simulink model "Syetem08"  (R2022b)
settings: Solver=ode45  StartTime=0.0  StopTime=Time  FixedStep=0.0001  RelTol=1e-6
values from neighbouring files (symbols this model uses):
  C1 = 2*M1*Wn1*zeta    [Syetem08_Parameters.m]
  C2 = 2*M2*Wn2*zeta    [Syetem08_Parameters.m]
  C3 = 2*M3*Wn3*zeta    [Syetem08_Parameters.m]
  dCD11 = 6.5*u    (= 6.5e-06)    [Syetem08_Parameters.m]
  dCD12 = 7.5*u    (= 7.5e-06)    [Syetem08_Parameters.m]
  dCD13 = 17*u    (= 1.7e-05)    [Syetem08_Parameters.m]
  dCD31 = dCD11    (= 6.5e-06)    [Syetem08_Parameters.m]
  dCD32 = dCD12    (= 7.5e-06)    [Syetem08_Parameters.m]
  dCD33 = dCD13    (= 1.7e-05)    [Syetem08_Parameters.m]
  epsilon = 8.854*u^2    (= 8.854e-12)    [Syetem08_Parameters.m]
  FAmp = -6*2*18*g    (= -2118.96)    [Syetem08_Parameters.m]
  g = 9.81    [Syetem08_Parameters.m]
  gCD1 = 5*u    (= 5e-06)    [Syetem08_Parameters.m]
  gCD3 = gCD1    (= 5e-06)    [Syetem08_Parameters.m]
  gppL1 = (14+.4)*u    (= 1.44e-05)    [Syetem08_Parameters.m]
  gppL12 = (20.5+.4+0.7+inaccuracy)*u    (= 2.21e-05)    [Syetem08_Parameters.m]
  gppL2 = (7+.4+inaccuracy)*u    (= 7.9e-06)    [Syetem08_Parameters.m]
  gppL3 = (7+.4-1.1+.1)*u    (= 6.4e-06)    [Syetem08_Parameters.m]
  gppL32 = (20.5+.4+0.7+inaccuracy)*u    (= 2.21e-05)    [Syetem08_Parameters.m]
  gppU1 = (7+.4-1.1+.2)*u    (= 6.5e-06)    [Syetem08_Parameters.m]
  gppU12 = (11.5+.4-0.7-inaccuracy)*u    (= 1.07e-05)    [Syetem08_Parameters.m]
  gppU2 = (7+.4-inaccuracy)*u    (= 6.9e-06)    [Syetem08_Parameters.m]
  gppU3 = (14+.4)*u    (= 1.44e-05)    [Syetem08_Parameters.m]
  gppU32 = (11.5+.4-0.7-inaccuracy)*u    (= 1.07e-05)    [Syetem08_Parameters.m]
  InputRatio = 0.814    [Syetem08_Parameters.m]
  K1 = 3*Kfactor*.9    (= 2.7)    [Syetem08_Parameters.m]
  K2 = 3*Kfactor*0.9    (= 2.7)    [Syetem08_Parameters.m]
  K3 = 3*Kfactor*.9    (= 2.7)    [Syetem08_Parameters.m]
  L1 = (215-.4)*u    (= 0.0002146)    [Syetem08_Parameters.m]
  L12 = (310-.4)*u    (= 0.0003096)    [Syetem08_Parameters.m]
  L2 = (215-.4)*u    (= 0.0002146)    [Syetem08_Parameters.m]
  L3 = (215-.4)*u    (= 0.0002146)    [Syetem08_Parameters.m]
  L32 = (310-.4)*u    (= 0.0003096)    [Syetem08_Parameters.m]
  M1 = rho*Depth*58910*u^2*Mfactor    (= 1.97654832e-07)    [Syetem08_Parameters.m]
  M2 = rho*Depth*75513.66*u^2*Mfactor    (= 2.53363432032e-07)    [Syetem08_Parameters.m]
  M3 = M1    (= 1.97654832e-07)    [Syetem08_Parameters.m]
  N1 = 8    [Syetem08_Parameters.m]
  N12 = 6    [Syetem08_Parameters.m]
  N2 = 2*5    (= 10)    [Syetem08_Parameters.m]
  N3 = N1    (= 8)    [Syetem08_Parameters.m]
  N32 = 6    [Syetem08_Parameters.m]
  NCD1 = 25    [Syetem08_Parameters.m]
  NCD3 = NCD1    (= 25)    [Syetem08_Parameters.m]
  S1 = [-inf 4.4]*u    [Syetem08_Parameters.m]
  S2 = [-(4.9+inaccuracy) (4.9-inaccuracy)]*u    [Syetem08_Parameters.m]
  S3 = [-3.7 inf]*u    [Syetem08_Parameters.m]
  t1 = 50*u    (= 5e-05)    [Syetem08_Parameters.m]
  t2 = t1    (= 5e-05)    [Syetem08_Parameters.m]
  t3 = t1    (= 5e-05)    [Syetem08_Parameters.m]
  Vcd1 = Vm1    (= 8.5)    [Syetem08_Parameters.m]
  Vm1 = 8.5    [Syetem08_Parameters.m]
  Vm2 = 27.5    [Syetem08_Parameters.m]
  Vm3 = 8.6    [Syetem08_Parameters.m]
  Vpp1 = Vm1    (= 8.5)    [Syetem08_Parameters.m]
  Vpp2 = 0    [Syetem08_Parameters.m]
  Vpp3 = Vm3    (= 8.6)    [Syetem08_Parameters.m]
  wCD1 = 3.5*u    (= 3.5e-06)    [Syetem08_Parameters.m]
  WCD1 = 427.5*u    (= 0.0004275)    [Syetem08_Parameters.m]
  wCD3 = wCD1    (= 3.5e-06)    [Syetem08_Parameters.m]
  WCD3 = WCD1    (= 0.0004275)    [Syetem08_Parameters.m]
undefined symbols (not defined in the file or in its folder): sigbuilder_block
settings Model: Creator=mokour  LastModifiedBy=Megdadi
settings DataIOCC: SaveFormat=StructureWithTime
settings OptimizationCC: LifeSpan=inf
settings DebuggingCC: UnconnectedInputMsg=warning  UnconnectedOutputMsg=warning  UnconnectedLineMsg=warning  SFExecutionAtInitializationDiag=none  SFMachineParentedDataDiag=warning  ArithmeticOperatorsInVariantConditions=warning
settings HardwareCC: ProdBitPerSizeT=32  ProdBitPerPtrDiffT=32  ProdWordSize=32  ProdHWDeviceType=Specified
settings ModelReferenceCC: EnableRefExpFcnMdlSchedulingChecks=on
settings SFSimCC: CustomCodeUndefinedFunction=UseInterfaceOnly
settings RTWCC: DLArmComputeVersion=19.05
settings CodeAppCC: StateflowObjectComments=on

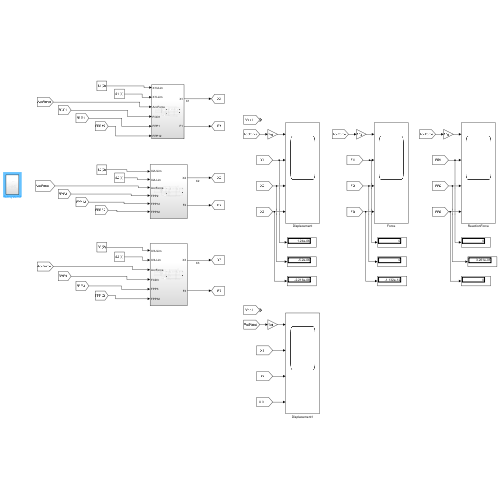
[thumbnail: Simulink's stored preview of the top-level diagram]
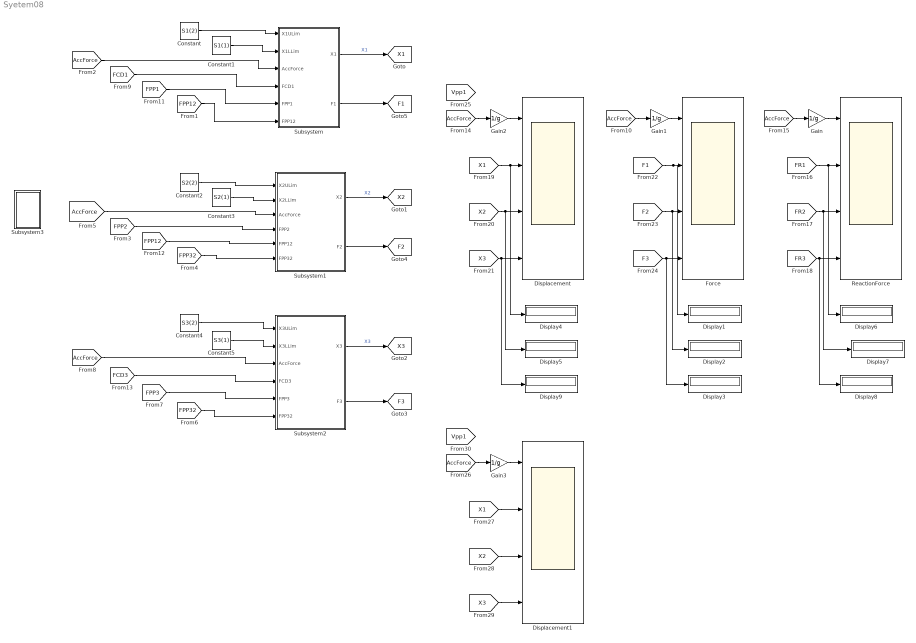
== system Syetem08 ==
  Constant : Constant  Value=S1(2)
  Constant1 : Constant  Value=S1(1)
  Constant2 : Constant  Value=S2(2)
  Constant3 : Constant  Value=S2(1)
  Constant4 : Constant  Value=S3(2)
  Constant5 : Constant  Value=S3(1)
  Displacement : Scope  NumInputPorts=4
  Displacement1 : Scope  NumInputPorts=4
  Display{1..9} (9 alike) : Display
  Force : Scope  NumInputPorts=4
  Gain{,1..3} (4 alike) : Gain  Gain=1/g
  ReactionForce : Scope  NumInputPorts=4
  Subsystem : Subsystem
  Subsystem1 : Subsystem
  Subsystem2 : Subsystem
  Subsystem3 : Subsystem
  tag scope: F1=global, F2=global, F3=global, X1=global, X2=global, X3=global
  wires:
  [FPP12] -> Subsystem/6(FPP12)
  [AccForce] -> Subsystem/3(AccForce)
  [FPP2] -> Subsystem1/4(FPP2)
  [FPP32] -> Subsystem1/6(FPP32)
  [AccForce] -> Subsystem1/3(AccForce)
  Subsystem1/1(X2) -> [X2]  "X2"
  Subsystem2/1(X3) -> [X3]  "X3"
  [FCD1] -> Subsystem/4(FCD1)
  [FPP1] -> Subsystem/5(FPP1)
  [FPP12] -> Subsystem1/5(FPP12)
  [FPP3] -> Subsystem2/5(FPP3)
  [FCD3] -> Subsystem2/4(FCD3)
  [AccForce] -> Subsystem2/3(AccForce)
  [FPP32] -> Subsystem2/6(FPP32)
  Subsystem2/2(F3) -> [F3]
  Subsystem/2(F1) -> [F1]
  Subsystem1/2(F2) -> [F2]
  Constant1/1 -> Subsystem/2(X1LLim)
  Constant/1 -> Subsystem/1(X1ULim)
  Constant3/1 -> Subsystem1/2(X2LLim)
  Constant2/1 -> Subsystem1/1(X2ULim)
  Constant4/1 -> Subsystem2/1(X3ULim)
  Constant5/1 -> Subsystem2/2(X3LLim)
  Gain/1 -> ReactionForce/1
  [FR1] -> ReactionForce/2, Display6/1
  [FR2] -> ReactionForce/3, Display7/1
  [FR3] -> ReactionForce/4, Display8/1
  Subsystem/1(X1) -> [X1]  "X1"
  [F3] -> Force/4, Display3/1
  [F2] -> Force/3, Display2/1
  [F1] -> Display1/1, Force/2
  [X1] -> Display4/1, Displacement/2
  [X2] -> Display5/1, Displacement/3
  [X3] -> Displacement/4, Display9/1
  [AccForce] -> Gain/1
  [AccForce] -> Gain1/1
  Gain1/1 -> Force/1
  [AccForce] -> Gain2/1
  Gain2/1 -> Displacement/1
  Gain3/1 -> Displacement1/1
  [AccForce] -> Gain3/1
  [X3] -> Displacement1/4
  [X2] -> Displacement1/3
  [X1] -> Displacement1/2

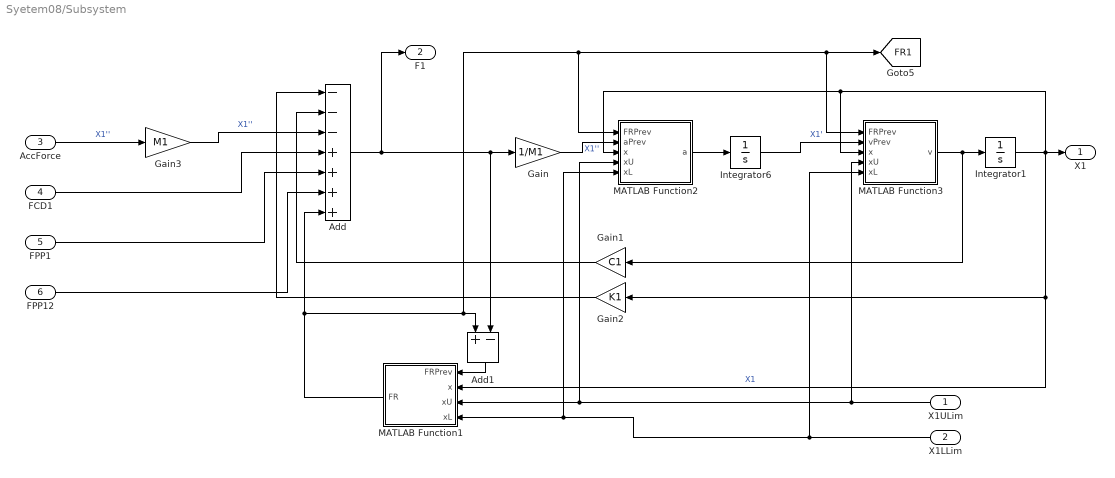
== system Syetem08/Subsystem ==
  X1ULim : Inport
  X1LLim : Inport  Port=2
  AccForce : Inport  Port=3
  FCD1 : Inport  Port=4
  FPP1 : Inport  Port=5
  FPP12 : Inport  Port=6
  Add : Sum  Inputs=---++++
  Add1 : Sum  Inputs=+-
  Gain : Gain  Gain=1/M1
  Gain1 : Gain  Gain=C1
  Gain2 : Gain  Gain=K1
  Gain3 : Gain  Gain=M1
  Integrator1 : Integrator  LimitOutput=on  UpperSaturationLimit=S1(2)  LowerSaturationLimit=S1(1)
  Integrator6 : Integrator  UpperSaturationLimit=0
  MATLAB Function1 : MATLAB Function  TreatAsAtomicUnit=on
  MATLAB Function2 : MATLAB Function  TreatAsAtomicUnit=on
  MATLAB Function3 : MATLAB Function  TreatAsAtomicUnit=on
  X1 : Outport
  F1 : Outport  Port=2
  tag scope: FR1=global
  wires:
  Gain3/1 -> Add/3  "X1''"
  FCD1/1 -> Add/4
  FPP1/1 -> Add/5
  FPP12/1 -> Add/6
  MATLAB Function1/1(FR) -> Add/7, MATLAB Function2/1(FRPrev), MATLAB Function3/1(FRPrev), [FR1], Add1/1
  Add1/1 -> MATLAB Function1/1(FRPrev)
  Gain2/1 -> Add/1
  Add/1 -> Add1/2, Gain/1, F1/1
  Gain1/1 -> Add/2
  Integrator1/1 -> X1/1, MATLAB Function3/3(x), MATLAB Function2/3(x), Gain2/1, MATLAB Function1/2(x)  "X1"
  Integrator6/1 -> MATLAB Function3/2(vPrev)  "X1'"
  X1ULim/1 -> MATLAB Function3/4(xU), MATLAB Function2/4(xU), MATLAB Function1/3(xU)
  X1LLim/1 -> MATLAB Function2/5(xL), MATLAB Function1/4(xL), MATLAB Function3/5(xL)
  MATLAB Function2/1(a) -> Integrator6/1
  Gain/1 -> MATLAB Function2/2(aPrev)  "X1''"
  MATLAB Function3/1(v) -> Gain1/1, Integrator1/1
  AccForce/1 -> Gain3/1  "X1''"

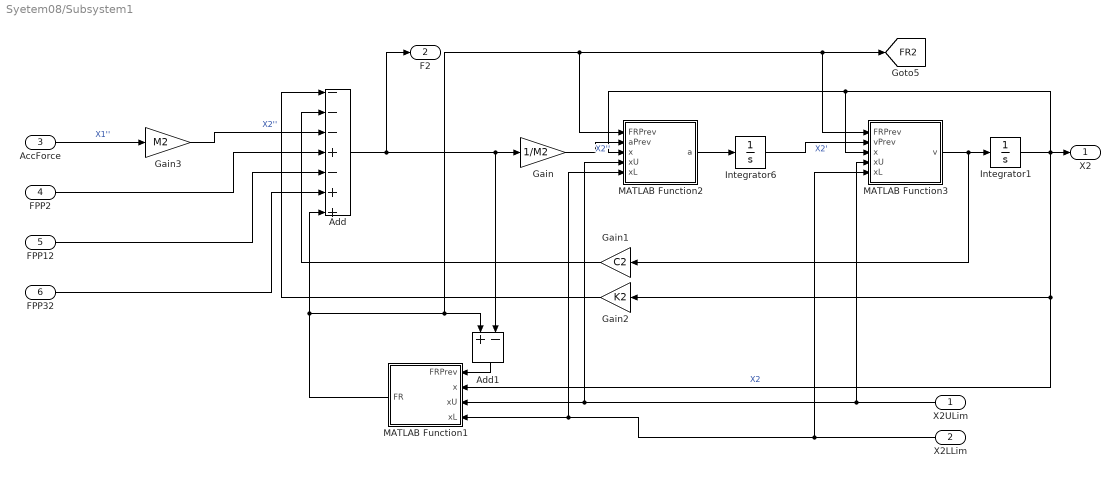
== system Syetem08/Subsystem1 ==
  X2ULim : Inport
  X2LLim : Inport  Port=2
  AccForce : Inport  Port=3
  FPP2 : Inport  Port=4
  FPP12 : Inport  Port=5
  FPP32 : Inport  Port=6
  Add : Sum  Inputs=---+-++
  Add1 : Sum  Inputs=+-
  Gain : Gain  Gain=1/M2
  Gain1 : Gain  Gain=C2
  Gain2 : Gain  Gain=K2
  Gain3 : Gain  Gain=M2
  Integrator1 : Integrator  LimitOutput=on  UpperSaturationLimit=S2(2)  LowerSaturationLimit=S2(1)
  Integrator6 : Integrator  UpperSaturationLimit=0
  MATLAB Function1 : MATLAB Function  TreatAsAtomicUnit=on
  MATLAB Function2 : MATLAB Function  TreatAsAtomicUnit=on
  MATLAB Function3 : MATLAB Function  TreatAsAtomicUnit=on
  X2 : Outport
  F2 : Outport  Port=2
  tag scope: FR2=global
  wires:
  FPP12/1 -> Add/5
  FPP2/1 -> Add/4
  FPP32/1 -> Add/6
  Gain3/1 -> Add/3  "X2''"
  Gain/1 -> MATLAB Function2/2(aPrev)  "X2''"
  X2ULim/1 -> MATLAB Function3/4(xU), MATLAB Function2/4(xU), MATLAB Function1/3(xU)
  Integrator6/1 -> MATLAB Function3/2(vPrev)  "X2'"
  Gain2/1 -> Add/1
  Gain1/1 -> Add/2
  X2LLim/1 -> MATLAB Function2/5(xL), MATLAB Function1/4(xL), MATLAB Function3/5(xL)
  MATLAB Function1/1(FR) -> Add/7, MATLAB Function2/1(FRPrev), MATLAB Function3/1(FRPrev), [FR2], Add1/1
  MATLAB Function3/1(v) -> Gain1/1, Integrator1/1
  Add1/1 -> MATLAB Function1/1(FRPrev)
  Add/1 -> Add1/2, Gain/1, F2/1
  MATLAB Function2/1(a) -> Integrator6/1
  AccForce/1 -> Gain3/1  "X1''"
  Integrator1/1 -> MATLAB Function3/3(x), MATLAB Function2/3(x), MATLAB Function1/2(x), Gain2/1, X2/1  "X2"

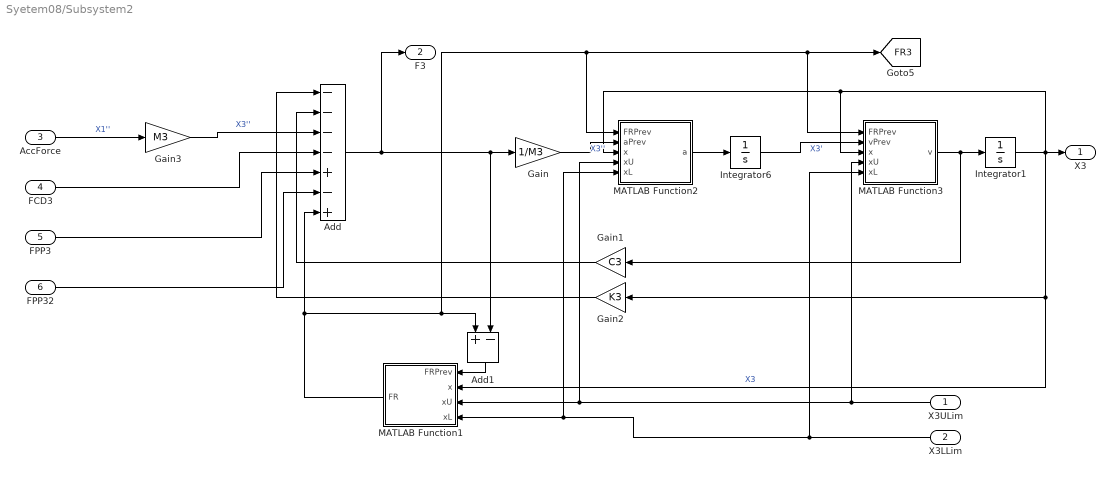
== system Syetem08/Subsystem2 ==
  X3ULim : Inport
  X3LLim : Inport  Port=2
  AccForce : Inport  Port=3
  FCD3 : Inport  Port=4
  FPP3 : Inport  Port=5
  FPP32 : Inport  Port=6
  Add : Sum  Inputs=----+-+
  Add1 : Sum  Inputs=+-
  Gain : Gain  Gain=1/M3
  Gain1 : Gain  Gain=C3
  Gain2 : Gain  Gain=K3
  Gain3 : Gain  Gain=M3
  Integrator1 : Integrator  LimitOutput=on  UpperSaturationLimit=S3(2)  LowerSaturationLimit=S3(1)
  Integrator6 : Integrator  UpperSaturationLimit=0
  MATLAB Function1 : MATLAB Function  TreatAsAtomicUnit=on
  MATLAB Function2 : MATLAB Function  TreatAsAtomicUnit=on
  MATLAB Function3 : MATLAB Function  TreatAsAtomicUnit=on
  X3 : Outport
  F3 : Outport  Port=2
  tag scope: FR3=global
  wires:
  FPP3/1 -> Add/5
  FCD3/1 -> Add/4
  FPP32/1 -> Add/6
  Gain3/1 -> Add/3  "X3''"
  Gain/1 -> MATLAB Function2/2(aPrev)  "X3''"
  X3ULim/1 -> MATLAB Function3/4(xU), MATLAB Function2/4(xU), MATLAB Function1/3(xU)
  Integrator6/1 -> MATLAB Function3/2(vPrev)  "X3'"
  Gain2/1 -> Add/1
  Gain1/1 -> Add/2
  X3LLim/1 -> MATLAB Function2/5(xL), MATLAB Function1/4(xL), MATLAB Function3/5(xL)
  MATLAB Function1/1(FR) -> Add/7, MATLAB Function2/1(FRPrev), MATLAB Function3/1(FRPrev), [FR3], Add1/1
  Add1/1 -> MATLAB Function1/1(FRPrev)
  Add/1 -> Add1/2, Gain/1, F3/1
  MATLAB Function2/1(a) -> Integrator6/1
  AccForce/1 -> Gain3/1  "X1''"
  Integrator1/1 -> MATLAB Function3/3(x), MATLAB Function2/3(x), Gain2/1, MATLAB Function1/2(x), X3/1  "X3"
  MATLAB Function3/1(v) -> Gain1/1, Integrator1/1

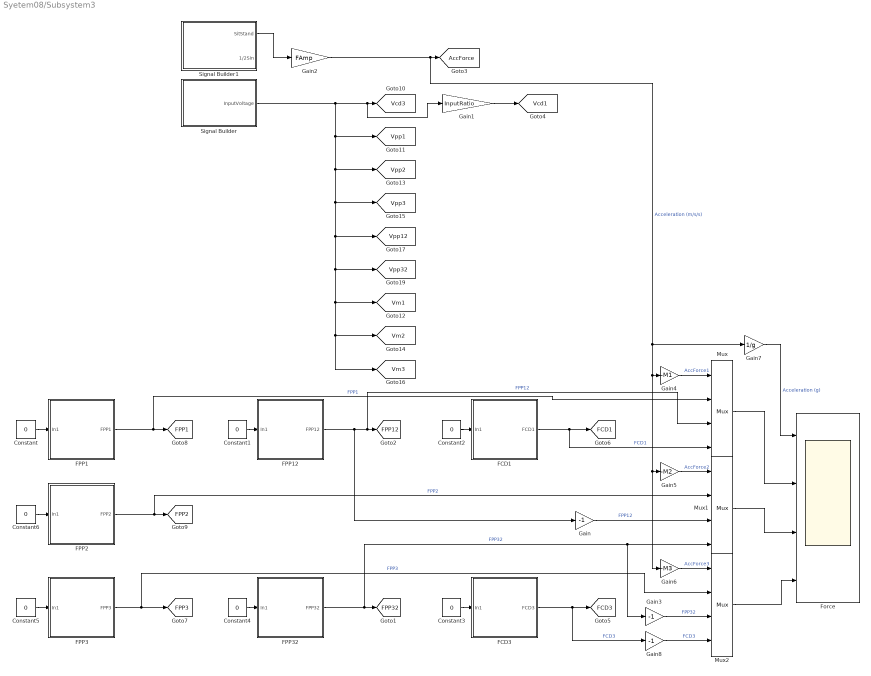
== system Syetem08/Subsystem3 ==
  Constant{,1..6} (7 alike) : Constant  Value=0
  FCD1 : Subsystem
  FCD3 : Subsystem
  FPP1 : Subsystem
  FPP12 : Subsystem
  FPP2 : Subsystem
  FPP3 : Subsystem
  FPP32 : Subsystem
  Force : Scope  NumInputPorts=4
  Gain : Gain  Gain=-1
  Gain1 : Gain  Gain=InputRatio
  Gain2 : Gain  Gain=FAmp
  Gain3 : Gain  Gain=-1
  Gain4 : Gain  Gain=-M1
  Gain5 : Gain  Gain=-M2
  Gain6 : Gain  Gain=-M3
  Gain7 : Gain  Gain=1/g
  Gain8 : Gain  Gain=-1
  Mux : Mux
  Mux1 : Mux
  Mux2 : Mux
  Signal Builder : Subsystem  Tag=STV Subsys  LoadFcn=sigbuilder_block('load');  StartFcn=sigbuilder_block('start');  StopFcn=sigbuilder_block('stop');  ClipboardFcn=sigbuilder_block('clipboard');  mask(Sigbuilder block){tuvar=[0:10]}
      mask help: Simulink:masks:SigbuilderBlock_MD
      mask init:
      | if ~strcmp(get_param(bdroot(gcbh),'SimulationStatus'),'stopped') tuvar = sigbuilder_block('maskInit'); end
      settings: CopyFcn=sigbuilder_block('copy');  DeleteFcn=sigbuilder_block('delete');  ModelCloseFcn=sigbuilder_block('modelClose');  PreSaveFcn=sigbuilder_block('preSave');  PauseFcn=sigbuilder_block('pause');  ContinueFcn=sigbuilder_block('continue');  NameChangeFcn=sigbuilder_block('namechange');  OpenFcn=sigbuilder_block('open',[437.6 153 550.4 359.25 ]);  CloseFcn=sigbuilder_block('close');
      mask Display: plot(0, 0, 100, 100,[2, 2, 32, 32, 2], [68, 8, 8, 68, 68],[32, 2], [38, 38], [32, 19, 2],[53, 60, 44], [32, 17, 17, 2],[16, 16, 31, 31]);txt = getActiveGroup(gcbh);text(2, 100, txt,'verticalAlignment', 'top');
  Signal Builder1 : Subsystem  Tag=STV Subsys  LoadFcn=sigbuilder_block('load');  StartFcn=sigbuilder_block('start');  StopFcn=sigbuilder_block('stop');  ClipboardFcn=sigbuilder_block('clipboard');  mask(Sigbuilder block){tuvar=[0:10]}
      mask help: Simulink:masks:SigbuilderBlock_MD
      mask init:
      | if ~strcmp(get_param(bdroot(gcbh),'SimulationStatus'),'stopped') tuvar = sigbuilder_block('maskInit'); end
      settings: CopyFcn=sigbuilder_block('copy');  DeleteFcn=sigbuilder_block('delete');  ModelCloseFcn=sigbuilder_block('modelClose');  PreSaveFcn=sigbuilder_block('preSave');  PauseFcn=sigbuilder_block('pause');  ContinueFcn=sigbuilder_block('continue');  NameChangeFcn=sigbuilder_block('namechange');  OpenFcn=sigbuilder_block('open',[6 77.25 1012.5 326.25 ]);  CloseFcn=sigbuilder_block('close');
      mask Display: plot(0, 0, 100, 100,[2, 2, 32, 32, 2], [68, 8, 8, 68, 68],[32, 2], [38, 38], [32, 19, 2],[53, 60, 44], [32, 17, 17, 2],[16, 16, 31, 31]);txt = getActiveGroup(gcbh);text(2, 100, txt,'verticalAlignment', 'top');
  tag scope: AccForce=global, FCD1=global, FCD3=global, FPP12=global, FPP1=global, FPP2=global, FPP32=global, FPP3=global, Vcd1=global, Vcd3=global, Vm1=global, Vm2=global, Vm3=global, Vpp12=global, Vpp1=global, Vpp2=global, Vpp32=global, Vpp3=global
  wires:
  FPP12/1(FPP12) -> Gain/1, Mux/3, [FPP12]  "FPP12"
  FPP32/1(FPP32) -> Mux1/4, Gain3/1, [FPP32]  "FPP32"
  FCD1/1(FCD1) -> Mux/4, [FCD1]  "FCD1"
  FCD3/1(FCD3) -> Gain8/1, [FCD3]  "FCD3"
  FPP3/1(FPP3) -> Mux2/2, [FPP3]  "FPP3"
  FPP1/1(FPP1) -> Mux/2, [FPP1]  "FPP1"
  FPP2/1(FPP2) -> Mux1/2, [FPP2]  "FPP2"
  Gain2/1 -> Gain6/1, Gain5/1, Gain4/1, Gain7/1, [AccForce]  "Acceleration (m/s/s)"
  Gain/1 -> Mux1/3  "FPP12"
  Gain3/1 -> Mux2/3  "FPP32"
  Gain4/1 -> Mux/1  "AccForce1"
  Gain5/1 -> Mux1/1  "AccForce2"
  Gain6/1 -> Mux2/1  "AccForce3"
  Mux/1 -> Force/2
  Mux1/1 -> Force/3
  Mux2/1 -> Force/4
  Gain7/1 -> Force/1  "Acceleration (g)"
  Gain1/1 -> [Vcd1]
  Gain8/1 -> Mux2/4  "FCD3"
  Constant/1 -> FPP1/1(In1)
  Constant1/1 -> FPP12/1(In1)
  Constant2/1 -> FCD1/1(In1)
  Constant3/1 -> FCD3/1(In1)
  Constant4/1 -> FPP32/1(In1)
  Constant5/1 -> FPP3/1(In1)
  Constant6/1 -> FPP2/1(In1)
  Signal Builder/1(InputVoltage) -> [Vm3], [Vm2], [Vm1], [Vpp32], [Vpp12], [Vpp3], [Vpp2], [Vpp1], Gain1/1, [Vcd3]
  Signal Builder1/1(SitStand) -> Gain2/1

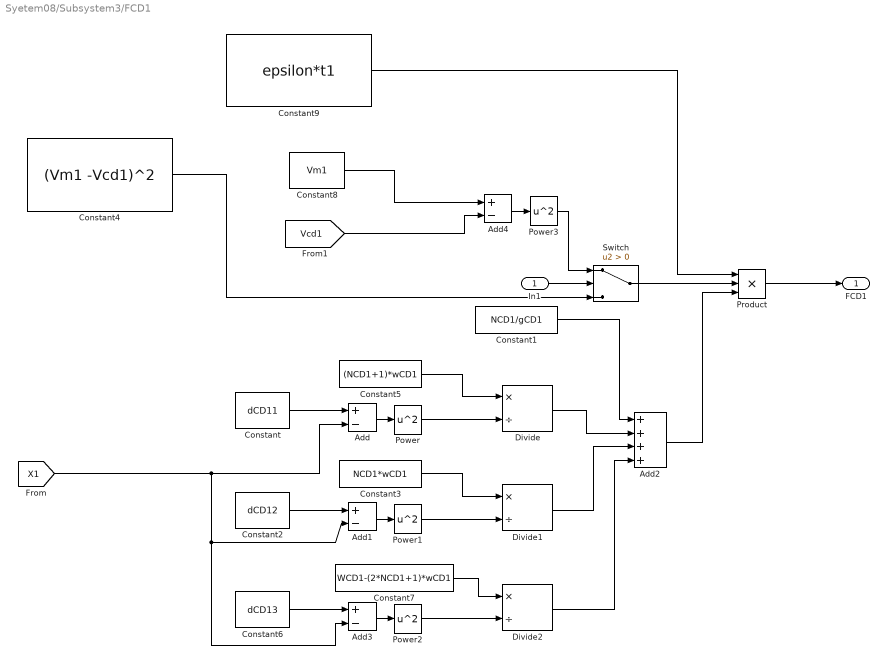
== system Syetem08/Subsystem3/FCD1 ==
  In1 : Inport
  Add{,1,3..4} (4 alike) : Sum  Inputs=+-
  Add2 : Sum  Inputs=++++
  Constant : Constant  Value=dCD11
  Constant1 : Constant  Value=NCD1/gCD1
  Constant2 : Constant  Value=dCD12
  Constant3 : Constant  Value=NCD1*wCD1
  Constant4 : Constant  Value=(Vm1 -Vcd1)^2
  Constant5 : Constant  Value=(NCD1+1)*wCD1
  Constant6 : Constant  Value=dCD13
  Constant7 : Constant  Value=WCD1-(2*NCD1+1)*wCD1
  Constant8 : Constant  Value=Vm1
  Constant9 : Constant  Value=epsilon*t1
  Divide : Product  Inputs=*/
  Divide1 : Product  Inputs=*/
  Divide2 : Product  Inputs=*/
  Power{,1..3} (4 alike) : Math  Operator=square  SignedPower=on
  Product : Product  Inputs=3
  Switch : Switch  Criteria=u2 > Threshold  SaturateOnIntegerOverflow=off  InputSameDT=off
  FCD1 : Outport
  wires:
  Constant1/1 -> Add2/1
  Power/1 -> Divide/2
  Add/1 -> Power/1
  Constant/1 -> Add/1
  Product/1 -> FCD1/1
  Add2/1 -> Product/3
  Constant5/1 -> Divide/1
  Divide/1 -> Add2/2
  Constant3/1 -> Divide1/1
  Constant2/1 -> Add1/1
  Add1/1 -> Power1/1
  Power1/1 -> Divide1/2
  Divide1/1 -> Add2/3
  Divide2/1 -> Add2/4
  Power2/1 -> Divide2/2
  Add3/1 -> Power2/1
  Constant6/1 -> Add3/1
  [X1] -> Add1/2, Add3/2, Add/2
  Constant7/1 -> Divide2/1
  Add4/1 -> Power3/1
  Constant8/1 -> Add4/1
  [Vcd1] -> Add4/2
  Constant9/1 -> Product/1
  Constant4/1 -> Switch/3
  Switch/1 -> Product/2
  Power3/1 -> Switch/1
  In1/1 -> Switch/2

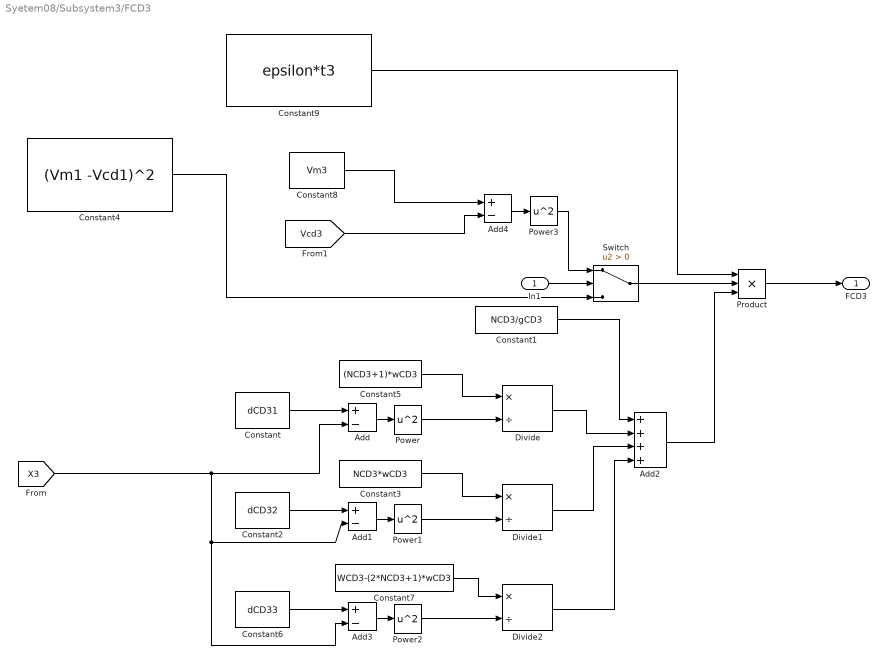
== system Syetem08/Subsystem3/FCD3 ==
  In1 : Inport
  Add{,1,3..4} (4 alike) : Sum  Inputs=+-
  Add2 : Sum  Inputs=++++
  Constant : Constant  Value=dCD31
  Constant1 : Constant  Value=NCD3/gCD3
  Constant2 : Constant  Value=dCD32
  Constant3 : Constant  Value=NCD3*wCD3
  Constant4 : Constant  Value=(Vm1 -Vcd1)^2
  Constant5 : Constant  Value=(NCD3+1)*wCD3
  Constant6 : Constant  Value=dCD33
  Constant7 : Constant  Value=WCD3-(2*NCD3+1)*wCD3
  Constant8 : Constant  Value=Vm3
  Constant9 : Constant  Value=epsilon*t3
  Divide : Product  Inputs=*/
  Divide1 : Product  Inputs=*/
  Divide2 : Product  Inputs=*/
  Power{,1..3} (4 alike) : Math  Operator=square  SignedPower=on
  Product : Product  Inputs=3
  Switch : Switch  Criteria=u2 > Threshold  SaturateOnIntegerOverflow=off  InputSameDT=off
  FCD3 : Outport
  wires:
  Constant7/1 -> Divide2/1
  [X3] -> Add/2, Add3/2, Add1/2
  Constant6/1 -> Add3/1
  Add3/1 -> Power2/1
  Power2/1 -> Divide2/2
  Divide2/1 -> Add2/4
  Divide1/1 -> Add2/3
  Power1/1 -> Divide1/2
  Add1/1 -> Power1/1
  Constant2/1 -> Add1/1
  Constant3/1 -> Divide1/1
  Divide/1 -> Add2/2
  Constant5/1 -> Divide/1
  Add2/1 -> Product/3
  Product/1 -> FCD3/1
  Constant/1 -> Add/1
  Add/1 -> Power/1
  Power/1 -> Divide/2
  Constant1/1 -> Add2/1
  Constant9/1 -> Product/1
  Add4/1 -> Power3/1
  [Vcd3] -> Add4/2
  Constant8/1 -> Add4/1
  Constant4/1 -> Switch/3
  Switch/1 -> Product/2
  Power3/1 -> Switch/1
  In1/1 -> Switch/2

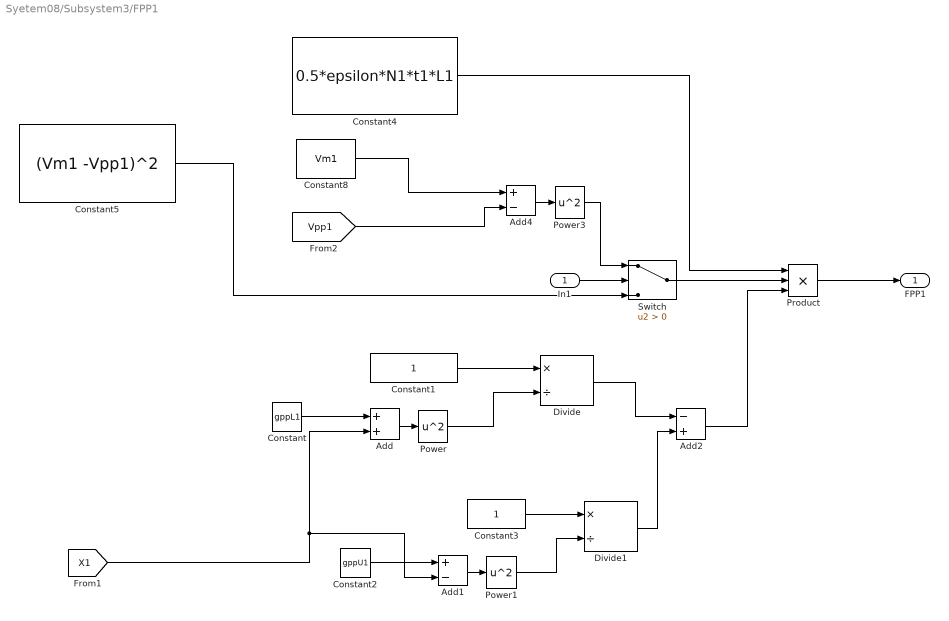
== system Syetem08/Subsystem3/FPP1 ==
  In1 : Inport
  Add : Sum
  Add1 : Sum  Inputs=+-
  Add2 : Sum  Inputs=-+
  Add4 : Sum  Inputs=+-
  Constant : Constant  Value=gppL1
  Constant1 : Constant
  Constant2 : Constant  Value=gppU1
  Constant3 : Constant
  Constant4 : Constant  Value=0.5*epsilon*N1*t1*L1
  Constant5 : Constant  Value=(Vm1 -Vpp1)^2
  Constant8 : Constant  Value=Vm1
  Divide : Product  Inputs=*/
  Divide1 : Product  Inputs=*/
  Power : Math  Operator=square  SignedPower=on
  Power1 : Math  Operator=square  SignedPower=on
  Power3 : Math  Operator=square  SignedPower=on
  Product : Product  Inputs=3
  Switch : Switch  Criteria=u2 > Threshold  SaturateOnIntegerOverflow=off  InputSameDT=off
  FPP1 : Outport
  wires:
  Constant3/1 -> Divide1/1
  Constant1/1 -> Divide/1
  Power/1 -> Divide/2
  Add/1 -> Power/1
  Add1/1 -> Power1/1
  Divide/1 -> Add2/1
  Constant2/1 -> Add1/1
  Constant/1 -> Add/1
  Power1/1 -> Divide1/2
  Product/1 -> FPP1/1
  Divide1/1 -> Add2/2
  [X1] -> Add/2, Add1/2
  Add2/1 -> Product/3
  Constant8/1 -> Add4/1
  Add4/1 -> Power3/1
  [Vpp1] -> Add4/2
  Constant4/1 -> Product/1
  Power3/1 -> Switch/1
  Constant5/1 -> Switch/3
  Switch/1 -> Product/2
  In1/1 -> Switch/2

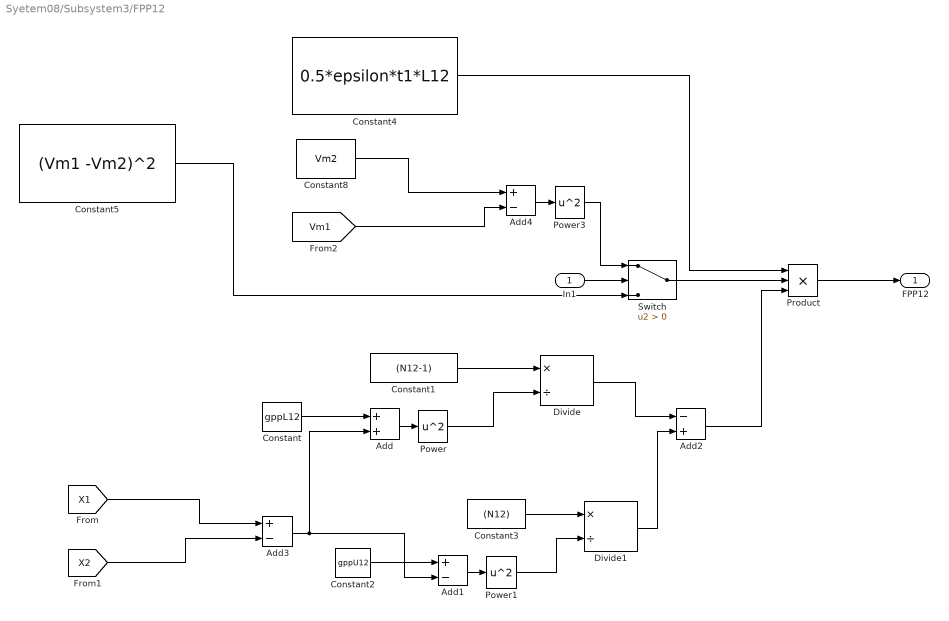
== system Syetem08/Subsystem3/FPP12 ==
  In1 : Inport
  Add : Sum
  Add1 : Sum  Inputs=+-
  Add2 : Sum  Inputs=-+
  Add3 : Sum  Inputs=+-
  Add4 : Sum  Inputs=+-
  Constant : Constant  Value=gppL12
  Constant1 : Constant  Value=(N12-1)
  Constant2 : Constant  Value=gppU12
  Constant3 : Constant  Value=(N12)
  Constant4 : Constant  Value=0.5*epsilon*t1*L12
  Constant5 : Constant  Value=(Vm1 -Vm2)^2
  Constant8 : Constant  Value=Vm2
  Divide : Product  Inputs=*/
  Divide1 : Product  Inputs=*/
  Power : Math  Operator=square  SignedPower=on
  Power1 : Math  Operator=square  SignedPower=on
  Power3 : Math  Operator=square  SignedPower=on
  Product : Product  Inputs=3
  Switch : Switch  Criteria=u2 > Threshold  SaturateOnIntegerOverflow=off  InputSameDT=off
  FPP12 : Outport
  wires:
  Constant3/1 -> Divide1/1
  Constant1/1 -> Divide/1
  Power/1 -> Divide/2
  Add/1 -> Power/1
  Add1/1 -> Power1/1
  Divide/1 -> Add2/1
  Constant2/1 -> Add1/1
  Constant/1 -> Add/1
  Power1/1 -> Divide1/2
  Product/1 -> FPP12/1
  Divide1/1 -> Add2/2
  Add2/1 -> Product/3
  [X1] -> Add3/1
  [X2] -> Add3/2
  Add3/1 -> Add/2, Add1/2
  Constant5/1 -> Switch/3
  Switch/1 -> Product/2
  Power3/1 -> Switch/1
  Constant8/1 -> Add4/1
  Add4/1 -> Power3/1
  [Vm1] -> Add4/2
  Constant4/1 -> Product/1
  In1/1 -> Switch/2

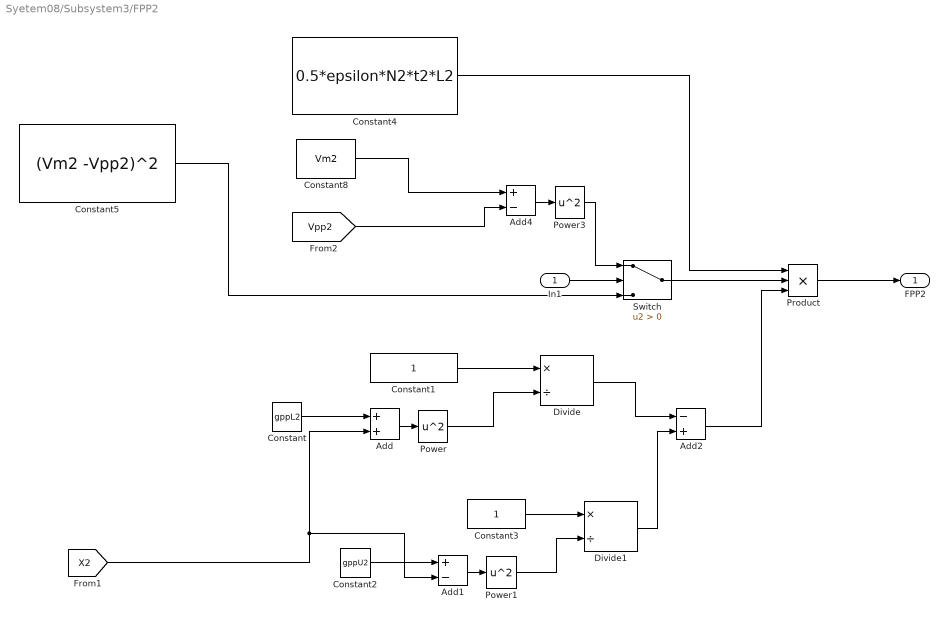
== system Syetem08/Subsystem3/FPP2 ==
  In1 : Inport
  Add : Sum
  Add1 : Sum  Inputs=+-
  Add2 : Sum  Inputs=-+
  Add4 : Sum  Inputs=+-
  Constant : Constant  Value=gppL2
  Constant1 : Constant
  Constant2 : Constant  Value=gppU2
  Constant3 : Constant
  Constant4 : Constant  Value=0.5*epsilon*N2*t2*L2
  Constant5 : Constant  Value=(Vm2 -Vpp2)^2
  Constant8 : Constant  Value=Vm2
  Divide : Product  Inputs=*/
  Divide1 : Product  Inputs=*/
  Power : Math  Operator=square  SignedPower=on
  Power1 : Math  Operator=square  SignedPower=on
  Power3 : Math  Operator=square  SignedPower=on
  Product : Product  Inputs=3
  Switch : Switch  Criteria=u2 > Threshold  SaturateOnIntegerOverflow=off  InputSameDT=off
  FPP2 : Outport
  wires:
  [X2] -> Add1/2, Add/2
  Add2/1 -> Product/3
  Divide1/1 -> Add2/2
  Product/1 -> FPP2/1
  Power1/1 -> Divide1/2
  Constant/1 -> Add/1
  Constant2/1 -> Add1/1
  Divide/1 -> Add2/1
  Add1/1 -> Power1/1
  Add/1 -> Power/1
  Power/1 -> Divide/2
  Constant1/1 -> Divide/1
  Constant3/1 -> Divide1/1
  Constant8/1 -> Add4/1
  Add4/1 -> Power3/1
  [Vpp2] -> Add4/2
  Constant4/1 -> Product/1
  Constant5/1 -> Switch/3
  Switch/1 -> Product/2
  Power3/1 -> Switch/1
  In1/1 -> Switch/2

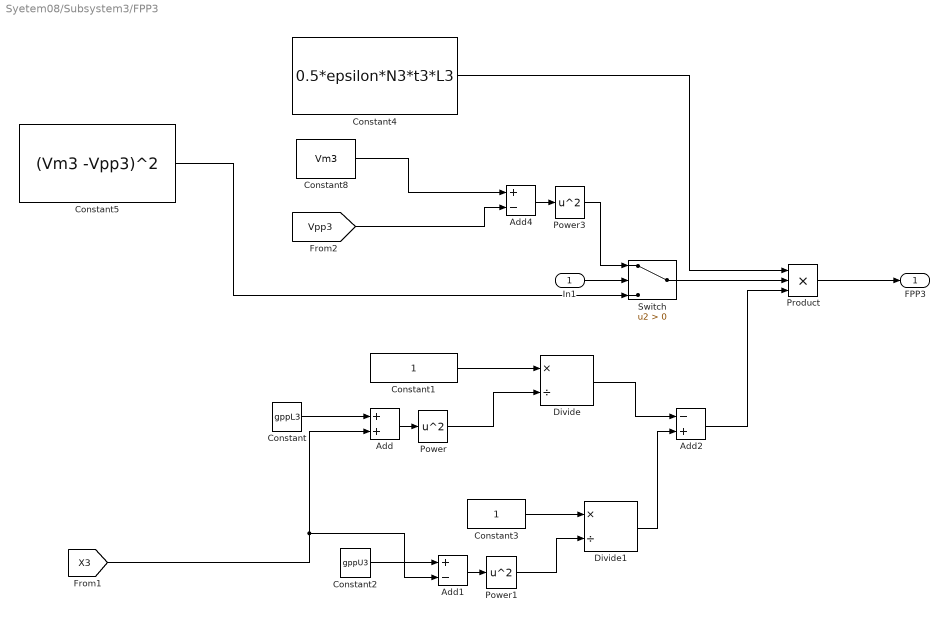
== system Syetem08/Subsystem3/FPP3 ==
  In1 : Inport
  Add : Sum
  Add1 : Sum  Inputs=+-
  Add2 : Sum  Inputs=-+
  Add4 : Sum  Inputs=+-
  Constant : Constant  Value=gppL3
  Constant1 : Constant
  Constant2 : Constant  Value=gppU3
  Constant3 : Constant
  Constant4 : Constant  Value=0.5*epsilon*N3*t3*L3
  Constant5 : Constant  Value=(Vm3 -Vpp3)^2
  Constant8 : Constant  Value=Vm3
  Divide : Product  Inputs=*/
  Divide1 : Product  Inputs=*/
  Power : Math  Operator=square  SignedPower=on
  Power1 : Math  Operator=square  SignedPower=on
  Power3 : Math  Operator=square  SignedPower=on
  Product : Product  Inputs=3
  Switch : Switch  Criteria=u2 > Threshold  SaturateOnIntegerOverflow=off  InputSameDT=off
  FPP3 : Outport
  wires:
  Constant3/1 -> Divide1/1
  Constant1/1 -> Divide/1
  Power/1 -> Divide/2
  Add/1 -> Power/1
  Add1/1 -> Power1/1
  Divide/1 -> Add2/1
  Constant2/1 -> Add1/1
  Constant/1 -> Add/1
  Constant4/1 -> Product/1
  Power1/1 -> Divide1/2
  Product/1 -> FPP3/1
  Divide1/1 -> Add2/2
  Add2/1 -> Product/3
  [X3] -> Add/2, Add1/2
  Constant8/1 -> Add4/1
  Add4/1 -> Power3/1
  [Vpp3] -> Add4/2
  Constant5/1 -> Switch/3
  Switch/1 -> Product/2
  Power3/1 -> Switch/1
  In1/1 -> Switch/2

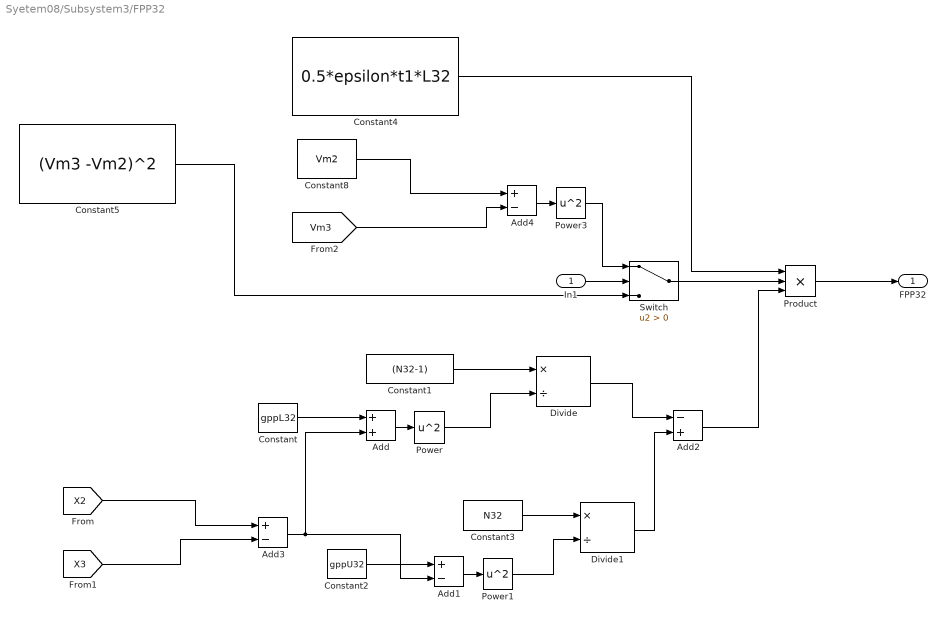
== system Syetem08/Subsystem3/FPP32 ==
  In1 : Inport
  Add : Sum
  Add1 : Sum  Inputs=+-
  Add2 : Sum  Inputs=-+
  Add3 : Sum  Inputs=+-
  Add4 : Sum  Inputs=+-
  Constant : Constant  Value=gppL32
  Constant1 : Constant  Value=(N32-1)
  Constant2 : Constant  Value=gppU32
  Constant3 : Constant  Value=N32
  Constant4 : Constant  Value=0.5*epsilon*t1*L32
  Constant5 : Constant  Value=(Vm3 -Vm2)^2
  Constant8 : Constant  Value=Vm2
  Divide : Product  Inputs=*/
  Divide1 : Product  Inputs=*/
  Power : Math  Operator=square  SignedPower=on
  Power1 : Math  Operator=square  SignedPower=on
  Power3 : Math  Operator=square  SignedPower=on
  Product : Product  Inputs=3
  Switch : Switch  Criteria=u2 > Threshold  SaturateOnIntegerOverflow=off  InputSameDT=off
  FPP32 : Outport
  wires:
  Add3/1 -> Add1/2, Add/2
  [X3] -> Add3/2
  [X2] -> Add3/1
  Add2/1 -> Product/3
  Divide1/1 -> Add2/2
  Product/1 -> FPP32/1
  Power1/1 -> Divide1/2
  Constant/1 -> Add/1
  Constant2/1 -> Add1/1
  Divide/1 -> Add2/1
  Add1/1 -> Power1/1
  Add/1 -> Power/1
  Power/1 -> Divide/2
  Constant1/1 -> Divide/1
  Constant3/1 -> Divide1/1
  [Vm3] -> Add4/2
  Add4/1 -> Power3/1
  Constant5/1 -> Switch/3
  Power3/1 -> Switch/1
  Switch/1 -> Product/2
  Constant4/1 -> Product/1
  Constant8/1 -> Add4/1
  In1/1 -> Switch/2

== system Syetem08/Subsystem3/Signal Builder ==
  Demux : Demux  Tag=STV Demux  Outputs=1
      settings: DisplayOption=none
  FromWs : FromWorkspace  Tag=STV FromWs  VariableName=tuvar  OutputAfterFinalValue=Holding final value
      SigBuilderData=|
      | common.afterFinalStr = 'Hold final value'
      | common.sampleTime = '0'
      | dataSet.timeRange = [0 1]
      | dataSet.name = 'Group 1'
      | sbobj.Groups.Name = 'Group 1'
      | sbobj.Groups.Signals.Name = 'InputVoltage'
      | sbobj.Groups.Signals.XData = [0 0.2 0.4 0.6 0.8 1]
      | sbobj.Groups.Signals.YData = [0 0 70 70 0 0]
      | sbobj.Groups.TimeRange = [0 1]
  InputVoltage : Outport  Tag=STV Outport
  wires:
  FromWs/1 -> Demux/1
  Demux/1 -> InputVoltage/1

== system Syetem08/Subsystem3/Signal Builder1 ==
  Demux : Demux  Tag=STV Demux  Outputs=2
      settings: DisplayOption=none
  FromWs : FromWorkspace  Tag=STV FromWs  VariableName=tuvar  OutputAfterFinalValue=Holding final value
      SigBuilderData=|
      | common.afterFinalStr = 'Hold final value'
      | common.sampleTime = '0'
      | dataSet.timeRange = [0 1]
      | dataSet.name = 'Group 1'
      | sbobj.Groups.Name = 'Group 1'
      | sbobj.Groups.Signals(1).Name = 'SitStand'
      | sbobj.Groups.Signals(1).XData = [0 0.2 0.3 0.4 0.8 1]
      | sbobj.Groups.Signals(1).YData = [0 0 1 -0.8 0 0]
      | sbobj.Groups.Signals(2).Name = '1/2Sin'
      | sbobj.Groups.Signals(2).XData = [0 0.1 0.2 0.3 0.4 0.5 0.6 0.7 0.8 0.9 1]
      | sbobj.Groups.Signals(2).YData = [0 0 0 0.70711 1 1 1 0.70711 0 0 0]
      | sbobj.Groups.TimeRange = [0 1]
  SitStand : Outport  Tag=STV Outport
  1/2Sin : Outport  Tag=STV Outport  Port=2
  wires:
  FromWs/1 -> Demux/1
  Demux/1 -> SitStand/1
  Demux/2 -> 1/2Sin/1

== matlab function Syetem08/Subsystem2/MATLAB Function3 ==
  data: FRPrev input; vPrev input; v output; x input; xU input; xL input
function v = fcn(FRPrev, vPrev, x, xU, xL)

if  (x >= xU && FRPrev < 0) || (x <= xL && FRPrev > 0)
    v = 0;
else
    v = vPrev;
end

end

== matlab function Syetem08/Subsystem2/MATLAB Function1 ==
  data: FRPrev input; FR output; x input; xU input; xL input
function FR = fcn(FRPrev, x, xU, xL)

if  (x >= xU && FRPrev < 0) || (x <= xL && FRPrev > 0)
    FR = FRPrev;
else
    FR = 0;
end

end

== matlab function Syetem08/Subsystem1/MATLAB Function1 ==
  data: FRPrev input; FR output; x input; xU input; xL input
function FR = fcn(FRPrev, x, xU, xL)

if  (x >= xU && FRPrev < 0) || (x <= xL && FRPrev > 0)
    FR = FRPrev;
else
    FR = 0;
end

end

== matlab function Syetem08/Subsystem1/MATLAB Function2 ==
  data: FRPrev input; aPrev input; a output; x input; xU input; xL input
function a = fcn(FRPrev, aPrev, x, xU, xL)

if  (x >= xU && FRPrev < 0) || (x <= xL && FRPrev > 0)
    a = 0;
else
    a = aPrev;
end

end

== matlab function Syetem08/Subsystem/MATLAB Function1 ==
  data: FRPrev input; FR output; x input; xU input; xL input
function FR = fcn(FRPrev, x, xU, xL)

if  (x >= xU && FRPrev < 0) || (x <= xL && FRPrev > 0)
    FR = FRPrev;
else
    FR = 0;
end

end

== matlab function Syetem08/Subsystem1/MATLAB Function3 ==
  data: FRPrev input; vPrev input; v output; x input; xU input; xL input
function v = fcn(FRPrev, vPrev, x, xU, xL)

if  (x >= xU && FRPrev < 0) || (x <= xL && FRPrev > 0)
    v = 0;
else
    v = vPrev;
end

end

== matlab function Syetem08/Subsystem/MATLAB Function2 ==
  data: FRPrev input; aPrev input; a output; x input; xU input; xL input
function a = fcn(FRPrev, aPrev, x, xU, xL)

if  (x >= xU && FRPrev < 0) || (x <= xL && FRPrev > 0)
    a = 0;
else
    a = aPrev;
end

end

== matlab function Syetem08/Subsystem/MATLAB Function3 ==
  data: FRPrev input; vPrev input; v output; x input; xU input; xL input
function v = fcn(FRPrev, vPrev, x, xU, xL)

if  (x >= xU && FRPrev < 0) || (x <= xL && FRPrev > 0)
    v = 0;
else
    v = vPrev;
end

end

== matlab function Syetem08/Subsystem2/MATLAB Function2 ==
  data: FRPrev input; aPrev input; a output; x input; xU input; xL input
function a = fcn(FRPrev, aPrev, x, xU, xL)

if  (x >= xU && FRPrev < 0) || (x <= xL && FRPrev > 0)
    a = 0;
else
    a = aPrev;
end

end
